simulink model "clearing_faulted_segment_travelling_Wave"  (R2018a)
settings: Solver=ode23t  StartTime=0.0  StopTime=2  MaxStep=1e-3  RelTol=1e-3
values from neighbouring files (symbols this model uses):
  AC_lim = [1.5 -1.5]    [MT_HVDC_initialize.m]
  C_pm = 10.48e-3    (= 0.01048)    [MT_HVDC_initialize.m]
  ccsc_lim = [1.0 -1.0]    [MT_HVDC_initialize.m]
  DC_lim = [1.05 -1.05]    [MT_HVDC_initialize.m]
  f = 50    [MT_HVDC_initialize.m]
  Fc = 50    [MT_HVDC_initialize.m]
  Fn_filter = 1000    [MT_HVDC_initialize.m]
  Ireg_lim_i = [1.5, -1.5]    [MT_HVDC_initialize.m]
  Ireg_lim_r = [1.5, -1.5]    [MT_HVDC_initialize.m]
  Ki_ACreg_i = 260    [MT_HVDC_initialize.m]
  Ki_ccsc = 5    [MT_HVDC_initialize.m]
  Ki_DCreg_r = 150    [MT_HVDC_initialize.m]
  Ki_Ireg_i = 200    [MT_HVDC_initialize.m]
  Ki_Ireg_r = 100    [MT_HVDC_initialize.m]
  Ki_R_inv = 150000    [MT_HVDC_initialize.m]
  Ki_R_rec = 5000    [MT_HVDC_initialize.m]
  Kp_ACreg_i = 2    [MT_HVDC_initialize.m]
  Kp_ccsc = 1    [MT_HVDC_initialize.m]
  Kp_DCreg_r = 8    [MT_HVDC_initialize.m]
  Kp_Ireg_i = 2    [MT_HVDC_initialize.m]
  Kp_Ireg_r = 2    [MT_HVDC_initialize.m]
  Kp_R_inv = 0.001    [MT_HVDC_initialize.m]
  Kp_R_rec = 0.001    [MT_HVDC_initialize.m]
  L1_pu = 0.109    [MT_HVDC_initialize.m]
  L2_pu = 0.0824    [MT_HVDC_initialize.m]
  L_arm = L_arm_pu*Z_base66/w    [MT_HVDC_initialize.m]
  L_arm_pu = 0.15    [MT_HVDC_initialize.m]
  L_int = X_int/w    [MT_HVDC_initialize.m]
  n = 50    [MT_HVDC_initialize.m]
  n2 = 50    [MT_HVDC_initialize.m]
  P_nom = 220e6    (= 220000000)    [MT_HVDC_initialize.m]
  R1_pu = 0.00206    [MT_HVDC_initialize.m]
  R2_pu = 0.00206    [MT_HVDC_initialize.m]
  R_arm = 0.03    [MT_HVDC_initialize.m]
  R_arm_pu = R_arm/Z_base66    [MT_HVDC_initialize.m]
  R_int = sqrt((z_int_400^2)/(1+xr_ratio^2))    [MT_HVDC_initialize.m]
  Rg_T1 = 40    [MT_HVDC_initialize.m]
  S1_nom = P_nom    (= 220000000)    [MT_HVDC_initialize.m]
  S2_nom = P_nom    (= 220000000)    [MT_HVDC_initialize.m]
  T_fault = 1.4    [MT_HVDC_initialize.m]
  Ts_Control = 40e-6    (= 4e-05)    [MT_HVDC_initialize.m]
  Ts_Power = 20e-6    (= 2e-05)    [MT_HVDC_initialize.m]
  V1_prim = V_prim    (= 400000)    [MT_HVDC_initialize.m]
  V1_sec = V_grid    (= 66000)    [MT_HVDC_initialize.m]
  V2_prim = V_grid    (= 66000)    [MT_HVDC_initialize.m]
  V2_sec = 18e3    (= 18000)    [MT_HVDC_initialize.m]
  V_ac_ref = 1.035    [MT_HVDC_initialize.m]
  V_grid = 66e3    (= 66000)    [MT_HVDC_initialize.m]
  V_prim = 400e3    (= 400000)    [MT_HVDC_initialize.m]
  Vc_pm_r = 0*Vdc_nom/n    (= 0)    [MT_HVDC_initialize.m]
  Vdc_nom = 135e3    (= 135000)    [MT_HVDC_initialize.m]
  w = 2*pi*f    (= 314.159265359)    [MT_HVDC_initialize.m]
  z0z1 = 0.8    [MT_HVDC_initialize.m]
  Zeta_filter = 1    [MT_HVDC_initialize.m]
undefined symbols (not defined in the file or in its folder): D1, Delta, DiscIntNeverNeededParam
libraries: powerlib x417, powerlib_meascontrol x130, simulink x84, powerlib_extras x8, simulink_extras x5
(part 1 of 17)
settings Model: SimulationMode=accelerator  NumberOfSteps=1000  SnapshotBufferSize=5000  SnapshotInterval=100  Creator=tslettba  LastModifiedBy=eslam
settings SolverCC: AlgebraicLoopSolver=LineSearch  DecoupledContinuousIntegration=on
settings OptimizationCC: BooleanDataType=off  EfficientMapNaN2IntZero=off
settings DebuggingCC: UnconnectedLineMsg=none
settings HardwareCC: TargetBitPerPointer=64  TargetBitPerSizeT=64  TargetBitPerPtrDiffT=64  TargetLongLongMode=on  TargetIntDivRoundTo=Zero  TargetEndianess=LittleEndian  TargetWordSize=64  TargetHWDeviceType=MATLAB Host  ProdEqTarget=off
settings ModelReferenceCC: ModelReferenceMinAlgLoopOccurrences=on
settings CodeAppCC: MaxIdLength=128
settings GRTTargetCC: TargetLangStandard=C89/C90 (ANSI)  CombineOutputUpdateFcns=off  GRTInterface=on
settings SimscapeCC: SimscapeNormalizeSystem=off

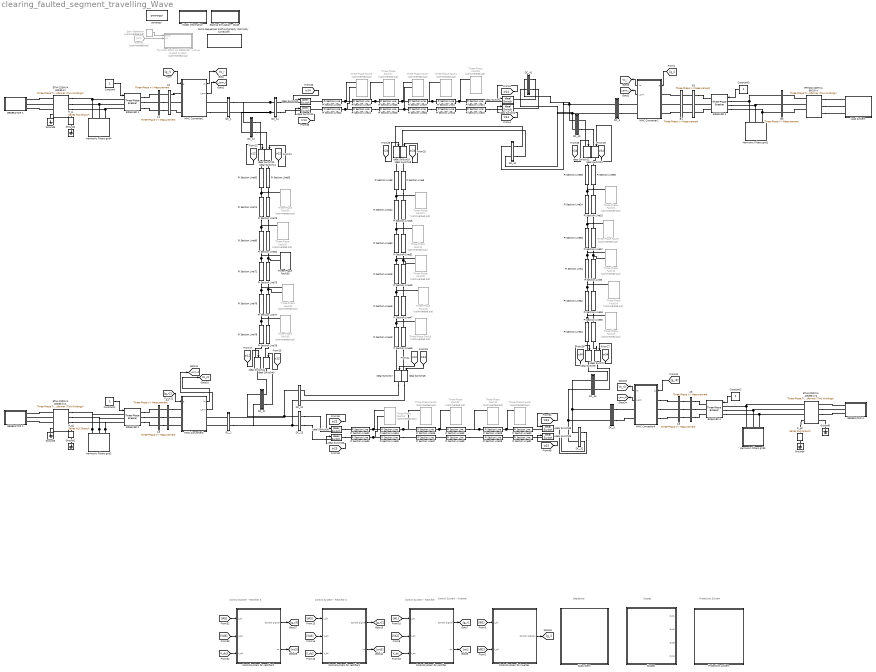
== system clearing_faulted_segment_travelling_Wave ==
  note: Protection System
  note: Scopes
  note: Control System - Inverter
  note: Control System - Rectifier
  note: Sequencer
  note: Control System - Rectifier 2
  note: Control System - Rectifier 3
  " " : powerlib_meascontrol/Pulse & Signal Generators/Stair Generator  Commented=on  t=[0, 999]  e=[1,0]  Ts=0
      settings: SourceProductName=Simscape Electrical
  " R_g" : powerlib/Elements/Series RLC Branch  LConnTagsString=__new0  RConnTagsString=__new0  BranchType=R  Resistance=Rg_T1  Inductance=1e-3  SetiL0=off  InitialCurrent=0  Capacitance=1e-6  Setx0=off  InitialVoltage=0  Measurements=None
      settings: SourceProductName=Simscape Electrical
  " R_g1" : powerlib/Elements/Series RLC Branch  LConnTagsString=__new0  RConnTagsString=__new0  BranchType=R  Resistance=Rg_T1  Inductance=1e-3  SetiL0=off  InitialCurrent=0  Capacitance=1e-6  Setx0=off  InitialVoltage=0  Measurements=None
      settings: SourceProductName=Simscape Electrical
  " R_g2" : powerlib/Elements/Series RLC Branch  LConnTagsString=__new0  RConnTagsString=__new0  BranchType=R  Resistance=Rg_T1  Inductance=1e-3  SetiL0=off  InitialCurrent=0  Capacitance=1e-6  Setx0=off  InitialVoltage=0  Measurements=None
      settings: SourceProductName=Simscape Electrical
  A1 : powerlib/Measurements/Three-Phase V-I Measurement  VoltageMeasurement=phase-to-phase  SetLabelV=on  LabelV=VA1  Vpu=off  VpuLL=off  CurrentMeasurement=yes  SetLabelI=on  LabelI=IA1  Ipu=off  Pbase=100e6  Vbase=500e3  OutputType=Complex  PhasorSimulation=off  PSBequivalent=0
      settings: SourceProductName=Simscape Electrical
  A2 : powerlib/Measurements/Three-Phase V-I Measurement  VoltageMeasurement=phase-to-ground  SetLabelV=on  LabelV=VA2  Vpu=off  VpuLL=off  CurrentMeasurement=no  SetLabelI=on  LabelI=IA2  Ipu=off  Pbase=100e6  Vbase=500e3  OutputType=Complex  PhasorSimulation=off  PSBequivalent=0
      settings: SourceProductName=Simscape Electrical
  A3 : powerlib/Measurements/Three-Phase V-I Measurement  VoltageMeasurement=phase-to-phase  SetLabelV=on  LabelV=VA3  Vpu=off  VpuLL=off  CurrentMeasurement=yes  SetLabelI=on  LabelI=IA3  Ipu=off  Pbase=100e6  Vbase=500e3  OutputType=Complex  PhasorSimulation=off  PSBequivalent=0
      settings: SourceProductName=Simscape Electrical
  A4 : powerlib/Measurements/Three-Phase V-I Measurement  VoltageMeasurement=phase-to-ground  SetLabelV=on  LabelV=VA4  Vpu=off  VpuLL=off  CurrentMeasurement=no  SetLabelI=on  LabelI=IA2  Ipu=off  Pbase=100e6  Vbase=500e3  OutputType=Complex  PhasorSimulation=off  PSBequivalent=0
      settings: SourceProductName=Simscape Electrical
  A5 : powerlib/Measurements/Three-Phase V-I Measurement  VoltageMeasurement=phase-to-phase  SetLabelV=on  LabelV=VA5  Vpu=off  VpuLL=off  CurrentMeasurement=yes  SetLabelI=on  LabelI=IA5  Ipu=off  Pbase=100e6  Vbase=500e3  OutputType=Complex  PhasorSimulation=off  PSBequivalent=0
      settings: SourceProductName=Simscape Electrical
  A6 : powerlib/Measurements/Three-Phase V-I Measurement  VoltageMeasurement=phase-to-ground  SetLabelV=on  LabelV=VA6  Vpu=off  VpuLL=off  CurrentMeasurement=no  SetLabelI=on  LabelI=IA2  Ipu=off  Pbase=100e6  Vbase=500e3  OutputType=Complex  PhasorSimulation=off  PSBequivalent=0
      settings: SourceProductName=Simscape Electrical
  B1 : powerlib/Measurements/Three-Phase V-I Measurement  VoltageMeasurement=phase-to-phase  SetLabelV=on  LabelV=VB1  Vpu=off  VpuLL=off  CurrentMeasurement=yes  SetLabelI=on  LabelI=IB1  Ipu=off  Pbase=100e6  Vbase=500e3  OutputType=Complex  PhasorSimulation=off  PSBequivalent=0
      settings: SourceProductName=Simscape Electrical
  B2 : powerlib/Measurements/Three-Phase V-I Measurement  VoltageMeasurement=phase-to-ground  SetLabelV=on  LabelV=VB2  Vpu=off  VpuLL=off  CurrentMeasurement=no  SetLabelI=on  LabelI=IB1  Ipu=off  Pbase=100e6  Vbase=500e3  OutputType=Complex  PhasorSimulation=off  PSBequivalent=0
      settings: SourceProductName=Simscape Electrical
  B3 : powerlib/Measurements/Three-Phase V-I Measurement  VoltageMeasurement=phase-to-ground  SetLabelV=on  LabelV=VB3  Vpu=off  VpuLL=off  CurrentMeasurement=yes  SetLabelI=on  LabelI=IB3  Ipu=off  Pbase=100e6  Vbase=500e3  OutputType=Complex  PhasorSimulation=off  PSBequivalent=0
      settings: SourceProductName=Simscape Electrical
  BREAKER {1..4} (4 alike) : powerlib/Elements/Three-Phase Breaker  InitialState=closed  SwitchA=on  SwitchB=on  SwitchC=on  SwitchTimes=[30/60]*10000  External=on  BreakerResistance=0.001  SnubberResistance=1e6  SnubberCapacitance=inf  Measurements=None
      settings: SourceProductName=Simscape Electrical
  Constant{,1..3} (4 alike) : Constant
  Controlsystem for Inverter : Subsystem  Variant=on  VariantControl=Variant1  OverrideUsingVariant=Variant1
  Controlsystem for rectifier : Subsystem  Variant=on  VariantControl=Variant1  OverrideUsingVariant=Variant1
  Controlsystem for rectifier1 : Subsystem  Variant=on  VariantControl=Variant1  OverrideUsingVariant=Variant1
  Controlsystem for rectifier2 : Subsystem  Variant=on  VariantControl=Variant1  OverrideUsingVariant=Variant1
  DC_1 : Subsystem
  DC_12 : Subsystem
  DC_14 : Subsystem
  DC_2 : Subsystem
  DC_21 : Subsystem
  DC_23 : Subsystem
  DC_24 : Subsystem
  DC_3 : Subsystem
  DC_32 : Subsystem
  DC_34 : Subsystem
  DC_4 : Subsystem
  DC_41 : Subsystem
  DC_42 : Subsystem
  DC_43 : Subsystem
  ETH102 220MVA 66/18 kV : powerlib/Elements/Three-Phase Transformer (Two Windings)  Winding1Connection=Yn  Winding2Connection=Delta (D1)  CoreType=Three single-phase transformers  SetSaturation=off  Hysteresis=off  DataFile='hysteresis'  SetInitialFlux=off  Measurements=None  UNITS=pu  NominalPower=[S2_nom , f ]  Winding1=[V2_prim , R2_pu*0.5 , L2_pu*0.5]  Winding2=[V2_sec , R2_pu*0.5 , L2_pu*0.5]  Rm=500  Lm=500  L0=0.5  Saturation="[ 0,0  ;  0.005,1.2  ;  1.0,1.4 ]"  InitialFluxes=[ 0.8 , -0.8 , 0.7 ]  MoreParameters=off  BreakLoop=off  DataType=off  TransfoNumber=0
      settings: SourceProductName=Simscape Electrical
  ETH4 220MVA 400/66 kV : powerlib/Elements/Three-Phase Transformer (Two Windings)  Winding1Connection=Yn  Winding2Connection=Yn  CoreType=Three single-phase transformers  SetSaturation=off  Hysteresis=off  DataFile='hysteresis'  SetInitialFlux=off  Measurements=None  UNITS=pu  NominalPower=[S1_nom , f ]  Winding1=[V1_prim , R1_pu*0.5, L1_pu*0.5]  Winding2=[V1_sec , R1_pu*0.5, L1_pu*0.5]  Rm=500  Lm=500  L0=0.5  Saturation="[ 0,0  ;  0.005,1.2  ;  1.0,1.4 ]"  InitialFluxes=[ 0.8 , -0.8 , 0.7 ]  MoreParameters=off  BreakLoop=off  DataType=off  TransfoNumber=0
      settings: SourceProductName=Simscape Electrical
  ETH4 220MVA 400/66 kV1 : powerlib/Elements/Three-Phase Transformer (Two Windings)  Winding1Connection=Yn  Winding2Connection=Yn  CoreType=Three single-phase transformers  SetSaturation=off  Hysteresis=off  DataFile='hysteresis'  SetInitialFlux=off  Measurements=None  UNITS=pu  NominalPower=[S1_nom , f ]  Winding1=[V1_prim , R1_pu*0.5, L1_pu*0.5]  Winding2=[V1_sec , R1_pu*0.5, L1_pu*0.5]  Rm=500  Lm=500  L0=0.5  Saturation="[ 0,0  ;  0.005,1.2  ;  1.0,1.4 ]"  InitialFluxes=[ 0.8 , -0.8 , 0.7 ]  MoreParameters=off  BreakLoop=off  DataType=off  TransfoNumber=0
      settings: SourceProductName=Simscape Electrical
  ETH4 220MVA 400/66 kV2 : powerlib/Elements/Three-Phase Transformer (Two Windings)  Winding1Connection=Yn  Winding2Connection=Yn  CoreType=Three single-phase transformers  SetSaturation=off  Hysteresis=off  DataFile='hysteresis'  SetInitialFlux=off  Measurements=None  UNITS=pu  NominalPower=[S1_nom , f ]  Winding1=[V1_prim , R1_pu*0.5, L1_pu*0.5]  Winding2=[V1_sec , R1_pu*0.5, L1_pu*0.5]  Rm=500  Lm=500  L0=0.5  Saturation="[ 0,0  ;  0.005,1.2  ;  1.0,1.4 ]"  InitialFluxes=[ 0.8 , -0.8 , 0.7 ]  MoreParameters=off  BreakLoop=off  DataType=off  TransfoNumber=0
      settings: SourceProductName=Simscape Electrical
  Extra Sequences and functionality (Normally turned off) : Subsystem
  From11 : From  Commented=on  GotoTag=wt
  GENERATOR 1 : Subsystem  mask{V_g=V_prim*1.03, F_s=f, R=R_int, L=L_int, T1=9999, T2=0.075, A=-0.5, BC=-0.5}
      mask prompts: V_g "Voltage (line-line RMS)"; F_s "Frequency:"; R "Internal Resistance:"; L "Internal inductance:"; T1 "Fault start:"; T2 "Fault duration:"; A "Phase A magnitude change:"; BC "Phase B,C magnitude change:"
      mask DialogControl DescTextVar Prompt: This block simulates a fully controllable Grid equivalent with internal parameters. It is possible to program voltage dips/swells for one, two or three phases.
      mask DialogControl asd Prompt: Source parameters:
      mask DialogControl Control3 Prompt: Fault simulation:
  GENERATOR 2 : Subsystem  mask{V_g=V_prim*1.03, F_s=f, R=R_int, L=L_int, T1=9999, T2=0.075, A=-0.5, BC=-0.5}
      mask prompts: V_g "Voltage (line-line RMS)"; F_s "Frequency:"; R "Internal Resistance:"; L "Internal inductance:"; T1 "Fault start:"; T2 "Fault duration:"; A "Phase A magnitude change:"; BC "Phase B,C magnitude change:"
      mask DialogControl DescTextVar Prompt: This block simulates a fully controllable Grid equivalent with internal parameters. It is possible to program voltage dips/swells for one, two or three phases.
      mask DialogControl asd Prompt: Source parameters:
      mask DialogControl Control3 Prompt: Fault simulation:
  GENERATOR 3 : Subsystem  mask{V_g=V_prim*1.03, F_s=f, R=R_int, L=L_int, T1=9999, T2=0.075, A=-0.5, BC=-0.5}
      mask prompts: V_g "Voltage (line-line RMS)"; F_s "Frequency:"; R "Internal Resistance:"; L "Internal inductance:"; T1 "Fault start:"; T2 "Fault duration:"; A "Phase A magnitude change:"; BC "Phase B,C magnitude change:"
      mask DialogControl DescTextVar Prompt: This block simulates a fully controllable Grid equivalent with internal parameters. It is possible to program voltage dips/swells for one, two or three phases.
      mask DialogControl asd Prompt: Source parameters:
      mask DialogControl Control3 Prompt: Fault simulation:
  Ground{1..6} (6 alike) : powerlib/Elements/Ground  LConnTagsString=a
      settings: SourceProductName=Simscape Electrical
  Harmonic Filters grid1 : Subsystem
      mask Display: disp('Harmonic Filters')
  Harmonic Filters grid2 : Subsystem
      mask Display: disp('Harmonic Filters')
  Harmonic Filters grid3 : Subsystem
      mask Display: disp('Harmonic Filters')
  Harmonic Filters grid4 : Subsystem
      mask Display: disp('Harmonic Filters')
  Ideal Switch{2,4,7,9..11,14..20,23,29..30,33,38,40..41} (20 alike) : powerlib/Power Electronics/Ideal Switch  Ron=0.001  Lon=0  IC=1  Rs=1e5  Cs=inf  Measurements=off
      settings: SourceProductName=Simscape Electrical
  Load System : Subsystem
      mask Display: disp('Load')
  MMC Converter1 : Subsystem
  MMC Converter2 : Subsystem
  MMC Converter3 : Subsystem
  MMC Converter4 : Subsystem
  Model Information : Subsystem
  Pi Section Line{1,4..5,8..11,14..15,18..39,44..59,72..84} (60 alike) : powerlib/Elements/Pi Section Line  LConnTagsString=__new0  RConnTagsString=__new0  Frequency=50  Resistance=0.01273  Inductance=0.9337e-3  Capacitance=12.74e-18  Length=25  PiSections=1  Measurements=None
      settings: AttributesFormatString=\n  SourceProductName=Simscape Electrical  SourceProductBaseCode=PS
  Protection system : Subsystem
  "Scopes " : Subsystem
  Startup Simulation - Guide : Subsystem
  Subsystem : Subsystem
  Three-Phase Fault{1,3,5,8..10,12..14,16..17,21..23,25} (15 alike) : powerlib/Elements/Three-Phase Fault  Commented=on  InitialStates=0  FaultA=on  FaultB=off  FaultC=off  GroundFault=on  SwitchTimes=0.7  External=off  SwitchStatus=NaN  FaultResistance=1  GroundResistance=1  SnubberResistance=1e6  SnubberCapacitance=inf  Measurements=Fault voltages and currents
      settings: SourceProductName=Simscape Electrical
  Three-Phase Fault15 : powerlib/Elements/Three-Phase Fault  Commented=on  InitialStates=0  FaultA=on  FaultB=off  FaultC=off  GroundFault=on  SwitchTimes=0.7  External=off  SwitchStatus=NaN  FaultResistance=0.1  GroundResistance=1  SnubberResistance=1e6  SnubberCapacitance=inf  Measurements=Fault voltages and currents
      settings: SourceProductName=Simscape Electrical
  Three-Phase Fault20 : powerlib/Elements/Three-Phase Fault  Commented=on  InitialStates=0  FaultA=off  FaultB=on  FaultC=off  GroundFault=on  SwitchTimes=0.7  External=off  SwitchStatus=NaN  FaultResistance=0.1  GroundResistance=1  SnubberResistance=1e6  SnubberCapacitance=inf  Measurements=Fault voltages and currents
      settings: SourceProductName=Simscape Electrical
  Three-Phase Fault24 : powerlib/Elements/Three-Phase Fault  Commented=on  InitialStates=0  FaultA=on  FaultB=off  FaultC=off  GroundFault=on  SwitchTimes=0.7  External=off  SwitchStatus=NaN  FaultResistance=0.1  GroundResistance=1  SnubberResistance=1e6  SnubberCapacitance=inf  Measurements=Fault voltages and currents
      settings: SourceProductName=Simscape Electrical
  Three-Phase Fault26 : powerlib/Elements/Three-Phase Fault  Commented=on  InitialStates=0  FaultA=on  FaultB=off  FaultC=off  GroundFault=on  SwitchTimes=1.5  External=off  SwitchStatus=NaN  FaultResistance=1  GroundResistance=1  SnubberResistance=1e6  SnubberCapacitance=inf  Measurements=Fault voltages and currents
      settings: SourceProductName=Simscape Electrical
  Three-Phase Fault32 : powerlib/Elements/Three-Phase Fault  Commented=on  InitialStates=0  FaultA=on  FaultB=off  FaultC=off  GroundFault=on  SwitchTimes=0.6  External=off  SwitchStatus=NaN  FaultResistance=0.1  GroundResistance=1  SnubberResistance=1e6  SnubberCapacitance=inf  Measurements=Fault voltages and currents
      settings: SourceProductName=Simscape Electrical
  Three-Phase Fault33 : powerlib/Elements/Three-Phase Fault  InitialStates=0  FaultA=on  FaultB=on  FaultC=off  GroundFault=on  SwitchTimes=1.5  External=off  SwitchStatus=NaN  FaultResistance=0.1  GroundResistance=1  SnubberResistance=1e6  SnubberCapacitance=inf  Measurements=Fault voltages and currents
      settings: SourceProductName=Simscape Electrical
  Three-Phase Fault34 : powerlib/Elements/Three-Phase Fault  Commented=on  InitialStates=0  FaultA=on  FaultB=off  FaultC=off  GroundFault=on  SwitchTimes=0.6  External=off  SwitchStatus=NaN  FaultResistance=1  GroundResistance=1  SnubberResistance=1e6  SnubberCapacitance=inf  Measurements=Fault voltages and currents
      settings: SourceProductName=Simscape Electrical
  Three-Phase Fault35 : powerlib/Elements/Three-Phase Fault  Commented=on  InitialStates=0  FaultA=on  FaultB=off  FaultC=off  GroundFault=on  SwitchTimes=0.6  External=off  SwitchStatus=NaN  FaultResistance=0.1  GroundResistance=1  SnubberResistance=1e6  SnubberCapacitance=inf  Measurements=Fault voltages and currents
      settings: SourceProductName=Simscape Electrical
  Three-Phase Fault6 : powerlib/Elements/Three-Phase Fault  Commented=on  InitialStates=0  FaultA=on  FaultB=off  FaultC=off  GroundFault=on  SwitchTimes=0.7  External=off  SwitchStatus=NaN  FaultResistance=0.1  GroundResistance=1  SnubberResistance=1e6  SnubberCapacitance=inf  Measurements=Fault voltages and currents
      settings: SourceProductName=Simscape Electrical
  Three-Phase Fault7 : powerlib/Elements/Three-Phase Fault  Commented=on  InitialStates=0  FaultA=off  FaultB=on  FaultC=off  GroundFault=on  SwitchTimes=0.6  External=off  SwitchStatus=NaN  FaultResistance=1  GroundResistance=1  SnubberResistance=1e6  SnubberCapacitance=inf  Measurements=Fault voltages and currents
      settings: SourceProductName=Simscape Electrical
  Thyristor Static AC BREAKER - Active bypass system : Subsystem  Commented=on
  powergui : powerlib/powergui  Priority=1  SimulationMode=Discrete  SampleTime=Ts_Power  frequency=60  Iterations=50  frequencyindice=0  Pbase=100e6  ErrMax=1e-4  UnitsV=kV  UnitsW=MW  buscounter=0  FunctionMessages=off  echomessages=off  EnableUseOfTLC=off  CurrentSourceSwitches=off  DisableSnubberDevices=off  DisableRonSwitches=off  DisableVfSwitches=off  DisplayEquations=off  SolverType=Tustin/Backward Euler (TBE)  Interpol=off  ExternalGateDelay=off  methode=off  Ts=100  x0status=blocks  SPID=on  SwTol=0  HookPort=off  RestoreLinks=warning  ResistiveCurrentMeasurement=off  Frange=[0:10:1000000]  Ylog=off  Xlog=on  ShowGrid=on  save=off  variable=ZData  structure=I_inv  ZoomFFT=off  StartTime=2  cycles=1  DisplayStyle=1  fundamental=50  FreqAxis=on  MaxFrequency=3000  frequencyindicesteady=1  RmsSteady=1  display=off
  tag scope: I_arm_i=global, I_arm_r2=global, I_arm_r3=global, I_arm_r=global, Vc_i=global, Vc_r2=global, Vc_r3=global, Vc_r=global
  wires:
  [g_i] -> MMC Converter2/1(g)
  MMC Converter1/1(Vc) -> [Vc_r]
  MMC Converter1/2(I_arm) -> [I_arm_r]
  MMC Converter2/2(I_arm) -> [I_arm_i]
  MMC Converter2/1(Vc) -> [Vc_i]
  [g_r] -> MMC Converter1/1(g)
  Controlsystem for Inverter/1(" Control Signal1") -> [g_i]
  [VB2] -> Controlsystem for Inverter/2("V_ph ")
  [IB1] -> Controlsystem for Inverter/1("I_ph ")
  [IA1] -> Controlsystem for rectifier/1("I_ph ")
  [VA2] -> Controlsystem for rectifier/2("V_ph ")
  [V_dc] -> Controlsystem for rectifier/3("V_dc ")
  Controlsystem for rectifier/1(" Control Signal") -> [g_r]
  " "/1 -> Thyristor Static AC BREAKER - Active bypass system/1(Block)
  Controlsystem for rectifier/2(" wt") -> [wt]
  From11/1 -> Thyristor Static AC BREAKER - Active bypass system/2(wt)
  Constant/1 -> BREAKER 1/1
  MMC Converter3/2(I_arm) -> [I_arm_r2]
  Constant1/1 -> BREAKER 2/1
  MMC Converter3/1(Vc) -> [Vc_r2]
  [g_r2] -> MMC Converter3/1(g)
  [IA3] -> Controlsystem for rectifier1/1("I_ph ")
  [VA4] -> Controlsystem for rectifier1/2("V_ph ")
  [V_dc2] -> Controlsystem for rectifier1/3("V_dc ")
  Controlsystem for rectifier1/2(" wt") -> [wt2]
  Controlsystem for rectifier1/1(" Control Signal") -> [g_r2]
  Constant2/1 -> BREAKER 3/1
  [g_r3] -> MMC Converter4/1(g)
  MMC Converter4/2(I_arm) -> [I_arm_r3]
  MMC Converter4/1(Vc) -> [Vc_r3]
  Controlsystem for rectifier2/1(" Control Signal") -> [g_r3]
  Controlsystem for rectifier2/2(" wt") -> [wt3]
  [V_dc3] -> Controlsystem for rectifier2/3("V_dc ")
  [VA6] -> Controlsystem for rectifier2/2("V_ph ")
  [IA5] -> Controlsystem for rectifier2/1("I_ph ")
  Constant3/1 -> BREAKER 4/1
  [tr14] -> Ideal Switch2/1
  [tr34] -> Ideal Switch10/1
  [tr34] -> Ideal Switch11/1
  [tr14] -> Ideal Switch4/1
  [tr24] -> Ideal Switch18/1
  [tr34] -> Ideal Switch7/1
  [tr12] -> Ideal Switch14/1
  [tr24] -> Ideal Switch16/1
  [tr34] -> Ideal Switch9/1
  [tr12] -> Ideal Switch41/1
  [tr14] -> Ideal Switch23/1
  [tr23] -> Ideal Switch33/1
  [tr23] -> Ideal Switch30/1
  [tr24] -> Ideal Switch19/1
  [tr12] -> Ideal Switch15/1
  [tr23] -> Ideal Switch38/1
  [tr23] -> Ideal Switch29/1
  [tr14] -> Ideal Switch20/1
  [tr12] -> Ideal Switch40/1
  [tr24] -> Ideal Switch17/1
  connections:
  B2/LConn3 -- B1/RConn3
  B2/LConn2 -- B1/RConn2
  B2/LConn1 -- B1/RConn1
  DC_1/LConn1 -- MMC Converter1/RConn1
  B1/LConn3 -- MMC Converter2/LConn3
  BREAKER 1/RConn3 -- A1/LConn3
  BREAKER 1/RConn1 -- A1/LConn1
  BREAKER 1/RConn2 -- A1/LConn2
  A2/LConn1 -- A1/RConn1
  A1/RConn2 -- A2/LConn2
  A1/RConn3 -- A2/LConn3
  MMC Converter1/LConn3 -- A2/RConn3
  MMC Converter1/LConn2 -- A2/RConn2
  B3/LConn1 -- BREAKER 4/LConn1 -- Harmonic Filters grid1/LConn1
  B3/LConn3 -- BREAKER 4/LConn3 -- Harmonic Filters grid1/LConn3
  B3/LConn2 -- BREAKER 4/LConn2 -- Harmonic Filters grid1/LConn2
  ETH102 220MVA 66/18 kV/RConn1 -- Load System/LConn1
  ETH102 220MVA 66/18 kV/RConn3 -- Load System/LConn3
  ETH4 220MVA 400/66 kV/RConn3 -- BREAKER 1/LConn3 -- Harmonic Filters grid4/LConn3
  ETH4 220MVA 400/66 kV/RConn2 -- BREAKER 1/LConn2 -- Harmonic Filters grid4/LConn2
  ETH4 220MVA 400/66 kV/RConn1 -- BREAKER 1/LConn1 -- Harmonic Filters grid4/LConn1
  B1/LConn1 -- MMC Converter2/LConn1
  B1/LConn2 -- MMC Converter2/LConn2
  ETH102 220MVA 66/18 kV/RConn2 -- Load System/LConn2
  ETH102 220MVA 66/18 kV/LConn2 -- B3/RConn2
  ETH102 220MVA 66/18 kV/LConn3 -- B3/RConn3
  ETH102 220MVA 66/18 kV/LConn1 -- B3/RConn1
  ETH4 220MVA 400/66 kV/LConn2 -- GENERATOR 1/RConn2
  ETH4 220MVA 400/66 kV/LConn1 -- GENERATOR 1/RConn1
  ETH4 220MVA 400/66 kV/LConn3 -- GENERATOR 1/RConn3
  Ground2/LConn1 -- " R_g"/RConn1
  Ground5/LConn1 -- ETH4 220MVA 400/66 kV/LConn4
  ETH4 220MVA 400/66 kV/RConn4 -- " R_g"/LConn1
  A2/RConn1 -- MMC Converter1/LConn1
  Harmonic Filters grid2/LConn1 -- ETH4 220MVA 400/66 kV1/RConn1 -- BREAKER 2/LConn1
  Harmonic Filters grid2/LConn2 -- BREAKER 2/LConn2 -- ETH4 220MVA 400/66 kV1/RConn2
  Harmonic Filters grid2/LConn3 -- BREAKER 2/LConn3 -- ETH4 220MVA 400/66 kV1/RConn3
  MMC Converter3/LConn2 -- A4/RConn2
  ETH4 220MVA 400/66 kV1/LConn1 -- GENERATOR 2/RConn1
  BREAKER 2/RConn2 -- A3/LConn2
  A4/RConn1 -- MMC Converter3/LConn1
  ETH4 220MVA 400/66 kV1/LConn2 -- GENERATOR 2/RConn2
  Ground1/LConn1 -- " R_g1"/RConn1
  BREAKER 2/RConn3 -- A3/LConn3
  ETH4 220MVA 400/66 kV1/RConn4 -- " R_g1"/LConn1
  Ground3/LConn1 -- ETH4 220MVA 400/66 kV1/LConn4
  A3/RConn2 -- A4/LConn2
  ETH4 220MVA 400/66 kV1/LConn3 -- GENERATOR 2/RConn3
  BREAKER 2/RConn1 -- A3/LConn1
  A4/LConn1 -- A3/RConn1
  MMC Converter3/LConn3 -- A4/RConn3
  A3/RConn3 -- A4/LConn3
  Ground4/LConn1 -- " R_g2"/RConn1
  MMC Converter4/LConn1 -- A5/RConn1
  MMC Converter4/LConn2 -- A5/RConn2
  MMC Converter4/LConn3 -- A5/RConn3
  A6/LConn1 -- BREAKER 3/RConn1
  A6/LConn2 -- BREAKER 3/RConn2
  A6/LConn3 -- BREAKER 3/RConn3
  Harmonic Filters grid3/LConn1 -- ETH4 220MVA 400/66 kV2/RConn1 -- BREAKER 3/LConn1
  BREAKER 3/LConn2 -- ETH4 220MVA 400/66 kV2/RConn2 -- Harmonic Filters grid3/LConn2
  BREAKER 3/LConn3 -- Harmonic Filters grid3/LConn3 -- ETH4 220MVA 400/66 kV2/RConn3
  GENERATOR 3/RConn1 -- ETH4 220MVA 400/66 kV2/LConn1
  ETH4 220MVA 400/66 kV2/LConn2 -- GENERATOR 3/RConn2
  ETH4 220MVA 400/66 kV2/LConn3 -- GENERATOR 3/RConn3
  Ground6/LConn1 -- ETH4 220MVA 400/66 kV2/LConn4
  " R_g2"/LConn1 -- ETH4 220MVA 400/66 kV2/RConn4
  A5/LConn1 -- A6/RConn1
  A5/LConn2 -- A6/RConn2
  A5/LConn3 -- A6/RConn3
  DC_2/LConn2 -- MMC Converter3/RConn2
  DC_4/RConn2 -- MMC Converter2/RConn2
  MMC Converter1/RConn2 -- DC_1/LConn2
  DC_4/RConn1 -- MMC Converter2/RConn1
  DC_2/LConn1 -- MMC Converter3/RConn1
  DC_3/LConn1 -- MMC Converter4/RConn1
  DC_3/LConn2 -- MMC Converter4/RConn2
  B2/RConn1 -- BREAKER 4/RConn1
  BREAKER 4/RConn2 -- B2/RConn2
  BREAKER 4/RConn3 -- B2/RConn3
  Pi Section Line50/RConn1 -- Three-Phase Fault12/LConn1 -- Pi Section Line44/LConn1
  DC_14/LConn2 -- DC_12/LConn2 -- DC_1/RConn2
  Pi Section Line28/RConn1 -- Pi Section Line30/LConn1 -- Three-Phase Fault8/LConn1
  Pi Section Line4/RConn1 -- Three-Phase Fault15/LConn1 -- Pi Section Line56/LConn1
  Pi Section Line32/RConn1 -- Pi Section Line34/LConn1 -- Three-Phase Fault24/LConn1
  Pi Section Line73/RConn1 -- Three-Phase Fault33/LConn2 -- Pi Section Line81/LConn1
  Pi Section Line25/RConn1 -- Three-Phase Fault7/LConn1 -- Pi Section Line27/LConn1
  Pi Section Line21/RConn1 -- Three-Phase Fault6/LConn1 -- Pi Section Line23/LConn1
  Pi Section Line52/RConn1 -- Pi Section Line4/LConn1 -- Three-Phase Fault14/LConn1
  Pi Section Line33/RConn1 -- Pi Section Line35/LConn1 -- Three-Phase Fault24/LConn2
  Pi Section Line28/LConn1 -- Pi Section Line38/RConn1 -- Three-Phase Fault10/LConn1
  Pi Section Line22/RConn1 -- Pi Section Line24/LConn1 -- Three-Phase Fault6/LConn2
  DC_24/LConn2 -- DC_23/LConn2 -- DC_21/LConn2 -- DC_2/RConn2
  Pi Section Line36/RConn1 -- Pi Section Line38/LConn1 -- Three-Phase Fault25/LConn1
  Pi Section Line1/RConn1 -- Three-Phase Fault16/LConn1 -- Pi Section Line11/LConn1
  Pi Section Line76/RConn1 -- Pi Section Line72/LConn1 -- Three-Phase Fault32/LConn1
  Pi Section Line48/RConn1 -- Pi Section Line46/LConn1 -- Three-Phase Fault5/LConn1
  Pi Section Line54/RConn1 -- Three-Phase Fault23/LConn1 -- Pi Section Line52/LConn1
  Pi Section Line74/RConn1 -- Three-Phase Fault34/LConn1 -- Pi Section Line82/LConn1
  Pi Section Line34/RConn1 -- Three-Phase Fault9/LConn1 -- Pi Section Line36/LConn1
  DC_34/LConn2 -- DC_3/RConn2 -- DC_32/LConn2
  Pi Section Line23/RConn1 -- Pi Section Line25/LConn1 -- Three-Phase Fault17/LConn1
  Pi Section Line80/RConn1 -- Pi Section Line74/LConn1 -- Three-Phase Fault26/LConn1
  Pi Section Line46/RConn1 -- Three-Phase Fault13/LConn1 -- Pi Section Line18/LConn1
  DC_14/LConn1 -- DC_12/LConn1 -- DC_1/RConn1
  DC_24/LConn1 -- DC_23/LConn1 -- DC_2/RConn1 -- DC_21/LConn1
  DC_43/LConn1 -- DC_41/LConn1 -- DC_42/LConn1 -- DC_4/LConn1
  Pi Section Line56/RConn1 -- Pi Section Line14/LConn1 -- Three-Phase Fault3/LConn1
  Pi Section Line5/RConn1 -- Three-Phase Fault15/LConn2 -- Pi Section Line57/LConn1
  DC_43/LConn2 -- DC_41/LConn2 -- DC_42/LConn2 -- DC_4/LConn2
  Pi Section Line78/RConn1 -- Three-Phase Fault35/LConn1 -- Pi Section Line76/LConn1
  Pi Section Line72/RConn1 -- Three-Phase Fault33/LConn1 -- Pi Section Line80/LConn1
  Pi Section Line14/RConn1 -- Three-Phase Fault22/LConn1 -- Pi Section Line58/LConn1
  Pi Section Line1/LConn1 -- Pi Section Line27/RConn1 -- Three-Phase Fault1/LConn1
  Pi Section Line44/RConn1 -- Pi Section Line8/LConn1 -- Three-Phase Fault21/LConn1
  DC_3/RConn1 -- DC_34/LConn1 -- DC_32/LConn1
  Pi Section Line19/RConn1 -- Pi Section Line51/LConn1 -- Three-Phase Fault20/LConn2
  Pi Section Line18/RConn1 -- Pi Section Line50/LConn1 -- Three-Phase Fault20/LConn1
  Pi Section Line39/RConn1 -- Pi Section Line29/LConn1
  Pi Section Line35/RConn1 -- Pi Section Line37/LConn1
  Pi Section Line39/LConn1 -- Pi Section Line37/RConn1
  Ideal Switch29/LConn1 -- Pi Section Line31/RConn1
  Pi Section Line31/LConn1 -- Pi Section Line29/RConn1
  Pi Section Line84/RConn1 -- Pi Section Line10/LConn1
  Pi Section Line77/LConn1 -- Pi Section Line79/RConn1
  Ideal Switch11/LConn1 -- DC_43/RConn1
  DC_14/RConn1 -- Ideal Switch20/LConn1
  Pi Section Line83/LConn1 -- Pi Section Line75/RConn1
  Pi Section Line49/LConn1 -- Ideal Switch16/LConn1
  Ideal Switch17/LConn1 -- Pi Section Line48/LConn1
  Ideal Switch33/RConn1 -- Pi Section Line33/LConn1
  Ideal Switch16/RConn1 -- DC_24/RConn2
  Pi Section Line5/LConn1 -- Pi Section Line53/RConn1
  Pi Section Line24/RConn1 -- Pi Section Line26/LConn1
  Ideal Switch17/RConn1 -- DC_24/RConn1
  DC_41/RConn1 -- Ideal Switch4/RConn1
  Pi Section Line20/RConn1 -- Ideal Switch2/LConn1
  Pi Section Line47/LConn1 -- Pi Section Line49/RConn1
  Pi Section Line20/LConn1 -- Pi Section Line10/RConn1
  Pi Section Line78/LConn1 -- Ideal Switch41/LConn1
  DC_14/RConn2 -- Ideal Switch23/LConn1
  Pi Section Line15/LConn1 -- Pi Section Line57/RConn1
  DC_42/RConn2 -- Ideal Switch18/LConn1
  Pi Section Line73/LConn1 -- Three-Phase Fault32/LConn2 -- Pi Section Line77/RConn1
  Pi Section Line53/LConn1 -- Pi Section Line55/RConn1
  DC_32/RConn1 -- Ideal Switch38/RConn1
  Pi Section Line59/LConn1 -- Pi Section Line15/RConn1
  DC_23/RConn1 -- Ideal Switch30/LConn1
  Ideal Switch30/RConn1 -- Pi Section Line32/LConn1
  Pi Section Line58/RConn1 -- Ideal Switch11/RConn1
  Pi Section Line59/RConn1 -- Ideal Switch10/RConn1
  Ideal Switch7/LConn1 -- Pi Section Line55/LConn1
  DC_21/RConn1 -- Ideal Switch41/RConn1
  DC_32/RConn2 -- Ideal Switch29/RConn1
  Pi Section Line45/LConn1 -- Pi Section Line51/RConn1
  Pi Section Line9/RConn1 -- Ideal Switch18/RConn1
  DC_41/RConn2 -- Ideal Switch2/RConn1
  Pi Section Line22/LConn1 -- Ideal Switch23/RConn1
  Ideal Switch7/RConn1 -- DC_34/RConn2
  Pi Section Line8/RConn1 -- Ideal Switch19/RConn1
  Ideal Switch38/LConn1 -- Pi Section Line30/RConn1
  DC_42/RConn1 -- Ideal Switch19/LConn1
  Ideal Switch40/LConn1 -- Pi Section Line79/LConn1
  Pi Section Line11/RConn1 -- Ideal Switch4/LConn1
  DC_23/RConn2 -- Ideal Switch33/LConn1
  Pi Section Line21/LConn1 -- Ideal Switch20/RConn1
  Ideal Switch9/LConn1 -- Pi Section Line54/LConn1
  Pi Section Line9/LConn1 -- Pi Section Line45/RConn1
  Ideal Switch9/RConn1 -- DC_34/RConn1
  Pi Section Line84/LConn1 -- Three-Phase Fault7/LConn2 -- Pi Section Line26/RConn1
  DC_12/RConn1 -- Ideal Switch15/LConn1
  DC_43/RConn2 -- Ideal Switch10/LConn1
  DC_12/RConn2 -- Ideal Switch14/LConn1
  Pi Section Line82/RConn1 -- Ideal Switch15/RConn1
  Pi Section Line75/LConn1 -- Pi Section Line81/RConn1
  Pi Section Line83/RConn1 -- Ideal Switch14/RConn1
  DC_21/RConn2 -- Ideal Switch40/RConn1
  Pi Section Line19/LConn1 -- Pi Section Line47/RConn1

== system clearing_faulted_segment_travelling_Wave/Controlsystem for Inverter ==
  note: Two modes of control:
      | Classical dq0 control
      | Dual sequence dq0 control - allowing negative sequence control
      | such as negative current injection for grid and load support
      | during unbalanced faults.
      |
      | TO CHANGE BETWEEN -> RIGHT CLICK ON THE CONTROL BLOCK OUTSIDE OF THIS SUBSYSTEM
      | -> VARIANT -> OVERRIDE USING
  "I_ph " : Inport
  "V_ph " : Inport  Port=2
  Dq0 Control : Subsystem  VariantControl=Variant1
  Dq0 control with Dual Synchronous Reference Frame (DSRF) : Subsystem  VariantControl=Variant
  " Control Signal1" : Outport

== system clearing_faulted_segment_travelling_Wave/Controlsystem for rectifier ==
  note: Two modes of control:
      | Classical dq0 control
      | Dual sequence dq0 control - allowing negative sequence control
      | such as negative current injection for grid and load support
      | during unbalanced faults.
      |
      | TO CHANGE BETWEEN -> RIGHT CLICK ON THE CONTROL BLOCK OUTSIDE OF THIS SUBSYSTEM
      | -> VARIANT -> OVERRIDE USING
  "I_ph " : Inport
  "V_ph " : Inport  Port=2
  "V_dc " : Inport  Port=3
  Dq0 Control : Subsystem  VariantControl=Variant1
  Dq0 Control with Dual Synchronous Reference Frame (DSRF) : Subsystem  VariantControl=Variant2
  " Control Signal" : Outport
  " wt" : Outport  Port=2

== system clearing_faulted_segment_travelling_Wave/Controlsystem for rectifier1 ==
  note: Two modes of control:
      | Classical dq0 control
      | Dual sequence dq0 control - allowing negative sequence control
      | such as negative current injection for grid and load support
      | during unbalanced faults.
      |
      | TO CHANGE BETWEEN -> RIGHT CLICK ON THE CONTROL BLOCK OUTSIDE OF THIS SUBSYSTEM
      | -> VARIANT -> OVERRIDE USING
  "I_ph " : Inport
  "V_ph " : Inport  Port=2
  "V_dc " : Inport  Port=3
  Dq0 Control : Subsystem  VariantControl=Variant1
  Dq0 Control with Dual Synchronous Reference Frame (DSRF) : Subsystem  VariantControl=Variant2
  " Control Signal" : Outport
  " wt" : Outport  Port=2

== system clearing_faulted_segment_travelling_Wave/Controlsystem for rectifier2 ==
  note: Two modes of control:
      | Classical dq0 control
      | Dual sequence dq0 control - allowing negative sequence control
      | such as negative current injection for grid and load support
      | during unbalanced faults.
      |
      | TO CHANGE BETWEEN -> RIGHT CLICK ON THE CONTROL BLOCK OUTSIDE OF THIS SUBSYSTEM
      | -> VARIANT -> OVERRIDE USING
  "I_ph " : Inport
  "V_ph " : Inport  Port=2
  "V_dc " : Inport  Port=3
  Dq0 Control : Subsystem  VariantControl=Variant1
  Dq0 Control with Dual Synchronous Reference Frame (DSRF) : Subsystem  VariantControl=Variant2
  " Control Signal" : Outport
  " wt" : Outport  Port=2

== system clearing_faulted_segment_travelling_Wave/DC_1 ==
  Current Measurement2 : powerlib/Measurements/Current Measurement  PhasorSimulation=off  OutputType=Complex  PSBequivalent=0
      settings: SourceProductName=Simscape Electrical
  Voltage Measurement1 : powerlib/Measurements/Voltage Measurement  PhasorSimulation=off  OutputType=Complex  PSBequivalent=0
      settings: SourceProductName=Simscape Electrical
  P : PMIOPort  Side=Left
  M : PMIOPort  Port=2  Side=Left
  p : PMIOPort  Port=3  Side=Right
  m : PMIOPort  Port=4  Side=Right
  tag scope: I_dc=global, V_dc=global
  wires:
  Voltage Measurement1/1 -> [V_dc]
  Current Measurement2/1 -> [I_dc]
  connections:
  Current Measurement2/LConn1 -- Voltage Measurement1/LConn1 -- P/RConn1
  Voltage Measurement1/LConn2 -- m/RConn1 -- M/RConn1
  Current Measurement2/RConn1 -- p/RConn1

== system clearing_faulted_segment_travelling_Wave/DC_12 ==
  Current Measurement1 : powerlib/Measurements/Current Measurement  PhasorSimulation=off  OutputType=Complex  PSBequivalent=0
      settings: SourceProductName=Simscape Electrical
  Current Measurement2 : powerlib/Measurements/Current Measurement  PhasorSimulation=off  OutputType=Complex  PSBequivalent=0
      settings: SourceProductName=Simscape Electrical
  Voltage Measurement1 : powerlib/Measurements/Voltage Measurement  PhasorSimulation=off  OutputType=Complex  PSBequivalent=0
      settings: SourceProductName=Simscape Electrical
  P : PMIOPort  Side=Left
  M : PMIOPort  Port=2  Side=Left
  p : PMIOPort  Port=3  Side=Right
  m : PMIOPort  Port=4  Side=Right
  tag scope: I0_dc12=global, I_dc12=global, V_dc12=global
  wires:
  Current Measurement2/1 -> [I_dc12]
  Voltage Measurement1/1 -> [V_dc12]
  Current Measurement1/1 -> [I0_dc12]
  connections:
  Voltage Measurement1/LConn1 -- Current Measurement2/LConn1 -- P/RConn1
  Voltage Measurement1/LConn2 -- M/RConn1 -- Current Measurement1/LConn1
  Current Measurement2/RConn1 -- p/RConn1
  Current Measurement1/RConn1 -- m/RConn1

== system clearing_faulted_segment_travelling_Wave/DC_14 ==
  Current Measurement1 : powerlib/Measurements/Current Measurement  PhasorSimulation=off  OutputType=Complex  PSBequivalent=0
      settings: SourceProductName=Simscape Electrical
  Current Measurement2 : powerlib/Measurements/Current Measurement  PhasorSimulation=off  OutputType=Complex  PSBequivalent=0
      settings: SourceProductName=Simscape Electrical
  Voltage Measurement1 : powerlib/Measurements/Voltage Measurement  PhasorSimulation=off  OutputType=Complex  PSBequivalent=0
      settings: SourceProductName=Simscape Electrical
  P : PMIOPort  Side=Left
  M : PMIOPort  Port=2  Side=Left
  p : PMIOPort  Port=3  Side=Right
  m : PMIOPort  Port=4  Side=Right
  tag scope: I0_dc14=global, I_dc14=global, V_dc14=global
  wires:
  Current Measurement2/1 -> [I_dc14]
  Voltage Measurement1/1 -> [V_dc14]
  Current Measurement1/1 -> [I0_dc14]
  connections:
  Voltage Measurement1/LConn1 -- Current Measurement2/LConn1 -- P/RConn1
  Voltage Measurement1/LConn2 -- Current Measurement1/LConn1 -- M/RConn1
  Current Measurement2/RConn1 -- p/RConn1
  Current Measurement1/RConn1 -- m/RConn1

== system clearing_faulted_segment_travelling_Wave/DC_2 ==
  Current Measurement2 : powerlib/Measurements/Current Measurement  PhasorSimulation=off  OutputType=Complex  PSBequivalent=0
      settings: SourceProductName=Simscape Electrical
  Voltage Measurement1 : powerlib/Measurements/Voltage Measurement  PhasorSimulation=off  OutputType=Complex  PSBequivalent=0
      settings: SourceProductName=Simscape Electrical
  P : PMIOPort  Side=Left
  M : PMIOPort  Port=2  Side=Left
  p : PMIOPort  Port=3  Side=Right
  m : PMIOPort  Port=4  Side=Right
  tag scope: I_dc2=global, V_dc2=global
  wires:
  Voltage Measurement1/1 -> [V_dc2]
  Current Measurement2/1 -> [I_dc2]
  connections:
  Voltage Measurement1/LConn1 -- Current Measurement2/LConn1 -- P/RConn1
  Voltage Measurement1/LConn2 -- M/RConn1 -- m/RConn1
  Current Measurement2/RConn1 -- p/RConn1

== system clearing_faulted_segment_travelling_Wave/DC_21 ==
  Current Measurement1 : powerlib/Measurements/Current Measurement  PhasorSimulation=off  OutputType=Complex  PSBequivalent=0
      settings: SourceProductName=Simscape Electrical
  Current Measurement2 : powerlib/Measurements/Current Measurement  PhasorSimulation=off  OutputType=Complex  PSBequivalent=0
      settings: SourceProductName=Simscape Electrical
  Voltage Measurement1 : powerlib/Measurements/Voltage Measurement  PhasorSimulation=off  OutputType=Complex  PSBequivalent=0
      settings: SourceProductName=Simscape Electrical
  P : PMIOPort  Side=Left
  M : PMIOPort  Port=2  Side=Left
  p : PMIOPort  Port=3  Side=Right
  m : PMIOPort  Port=4  Side=Right
  tag scope: I0_dc21=global, I_dc21=global, V_dc21=global
  wires:
  Current Measurement2/1 -> [I_dc21]
  Voltage Measurement1/1 -> [V_dc21]
  Current Measurement1/1 -> [I0_dc21]
  connections:
  Voltage Measurement1/LConn1 -- Current Measurement2/LConn1 -- P/RConn1
  Voltage Measurement1/LConn2 -- Current Measurement1/LConn1 -- M/RConn1
  Current Measurement2/RConn1 -- p/RConn1
  Current Measurement1/RConn1 -- m/RConn1

== system clearing_faulted_segment_travelling_Wave/DC_23 ==
  Current Measurement1 : powerlib/Measurements/Current Measurement  PhasorSimulation=off  OutputType=Complex  PSBequivalent=0
      settings: SourceProductName=Simscape Electrical
  Current Measurement2 : powerlib/Measurements/Current Measurement  PhasorSimulation=off  OutputType=Complex  PSBequivalent=0
      settings: SourceProductName=Simscape Electrical
  Voltage Measurement1 : powerlib/Measurements/Voltage Measurement  PhasorSimulation=off  OutputType=Complex  PSBequivalent=0
      settings: SourceProductName=Simscape Electrical
  P : PMIOPort  Side=Left
  M : PMIOPort  Port=2  Side=Left
  p : PMIOPort  Port=3  Side=Right
  m : PMIOPort  Port=4  Side=Right
  tag scope: I0_dc23=global, I_dc23=global, V_dc23=global
  wires:
  Current Measurement2/1 -> [I_dc23]
  Voltage Measurement1/1 -> [V_dc23]
  Current Measurement1/1 -> [I0_dc23]
  connections:
  Voltage Measurement1/LConn1 -- Current Measurement2/LConn1 -- P/RConn1
  Current Measurement1/RConn1 -- m/RConn1
  Current Measurement2/RConn1 -- p/RConn1
  Voltage Measurement1/LConn2 -- M/RConn1 -- Current Measurement1/LConn1

== system clearing_faulted_segment_travelling_Wave/DC_24 ==
  Current Measurement1 : powerlib/Measurements/Current Measurement  PhasorSimulation=off  OutputType=Complex  PSBequivalent=0
      settings: SourceProductName=Simscape Electrical
  Current Measurement2 : powerlib/Measurements/Current Measurement  PhasorSimulation=off  OutputType=Complex  PSBequivalent=0
      settings: SourceProductName=Simscape Electrical
  Voltage Measurement1 : powerlib/Measurements/Voltage Measurement  PhasorSimulation=off  OutputType=Complex  PSBequivalent=0
      settings: SourceProductName=Simscape Electrical
  P : PMIOPort  Side=Left
  M : PMIOPort  Port=2  Side=Left
  p : PMIOPort  Port=3  Side=Right
  m : PMIOPort  Port=4  Side=Right
  tag scope: I0_dc24=global, I_dc24=global, V_dc24=global
  wires:
  Current Measurement2/1 -> [I_dc24]
  Voltage Measurement1/1 -> [V_dc24]
  Current Measurement1/1 -> [I0_dc24]
  connections:
  Voltage Measurement1/LConn1 -- Current Measurement2/LConn1 -- P/RConn1
  Voltage Measurement1/LConn2 -- Current Measurement1/LConn1 -- M/RConn1
  Current Measurement2/RConn1 -- p/RConn1
  Current Measurement1/RConn1 -- m/RConn1

== system clearing_faulted_segment_travelling_Wave/DC_3 ==
  Current Measurement2 : powerlib/Measurements/Current Measurement  PhasorSimulation=off  OutputType=Complex  PSBequivalent=0
      settings: SourceProductName=Simscape Electrical
  Voltage Measurement1 : powerlib/Measurements/Voltage Measurement  PhasorSimulation=off  OutputType=Complex  PSBequivalent=0
      settings: SourceProductName=Simscape Electrical
  P : PMIOPort  Side=Left
  M : PMIOPort  Port=2  Side=Left
  p : PMIOPort  Port=3  Side=Right
  m : PMIOPort  Port=4  Side=Right
  tag scope: I_dc3=global, V_dc3=global
  wires:
  Voltage Measurement1/1 -> [V_dc3]
  Current Measurement2/1 -> [I_dc3]
  connections:
  Voltage Measurement1/LConn1 -- Current Measurement2/LConn1 -- P/RConn1
  Voltage Measurement1/LConn2 -- M/RConn1 -- m/RConn1
  Current Measurement2/RConn1 -- p/RConn1

== system clearing_faulted_segment_travelling_Wave/DC_32 ==
  Current Measurement1 : powerlib/Measurements/Current Measurement  PhasorSimulation=off  OutputType=Complex  PSBequivalent=0
      settings: SourceProductName=Simscape Electrical
  Current Measurement2 : powerlib/Measurements/Current Measurement  PhasorSimulation=off  OutputType=Complex  PSBequivalent=0
      settings: SourceProductName=Simscape Electrical
  Voltage Measurement1 : powerlib/Measurements/Voltage Measurement  PhasorSimulation=off  OutputType=Complex  PSBequivalent=0
      settings: SourceProductName=Simscape Electrical
  P : PMIOPort  Side=Left
  M : PMIOPort  Port=2  Side=Left
  p : PMIOPort  Port=3  Side=Right
  m : PMIOPort  Port=4  Side=Right
  tag scope: I0_dc32=global, I_dc32=global, V_dc32=global
  wires:
  Current Measurement2/1 -> [I_dc32]
  Voltage Measurement1/1 -> [V_dc32]
  Current Measurement1/1 -> [I0_dc32]
  connections:
  Voltage Measurement1/LConn1 -- Current Measurement2/LConn1 -- P/RConn1
  Voltage Measurement1/LConn2 -- Current Measurement1/LConn1 -- M/RConn1
  Current Measurement2/RConn1 -- p/RConn1
  Current Measurement1/RConn1 -- m/RConn1

== system clearing_faulted_segment_travelling_Wave/DC_34 ==
  Current Measurement1 : powerlib/Measurements/Current Measurement  PhasorSimulation=off  OutputType=Complex  PSBequivalent=0
      settings: SourceProductName=Simscape Electrical
  Current Measurement2 : powerlib/Measurements/Current Measurement  PhasorSimulation=off  OutputType=Complex  PSBequivalent=0
      settings: SourceProductName=Simscape Electrical
  Voltage Measurement1 : powerlib/Measurements/Voltage Measurement  PhasorSimulation=off  OutputType=Complex  PSBequivalent=0
      settings: SourceProductName=Simscape Electrical
  P : PMIOPort  Side=Left
  M : PMIOPort  Port=2  Side=Left
  p : PMIOPort  Port=3  Side=Right
  m : PMIOPort  Port=4  Side=Right
  tag scope: I0_dc34=global, I_dc34=global, V_dc34=global
  wires:
  Current Measurement2/1 -> [I_dc34]
  Voltage Measurement1/1 -> [V_dc34]
  Current Measurement1/1 -> [I0_dc34]
  connections:
  Voltage Measurement1/LConn1 -- Current Measurement2/LConn1 -- P/RConn1
  Voltage Measurement1/LConn2 -- Current Measurement1/LConn1 -- M/RConn1
  Current Measurement2/RConn1 -- p/RConn1
  Current Measurement1/RConn1 -- m/RConn1

== system clearing_faulted_segment_travelling_Wave/DC_4 ==
  Current Measurement2 : powerlib/Measurements/Current Measurement  PhasorSimulation=off  OutputType=Complex  PSBequivalent=0
      settings: SourceProductName=Simscape Electrical
  Voltage Measurement1 : powerlib/Measurements/Voltage Measurement  PhasorSimulation=off  OutputType=Complex  PSBequivalent=0
      settings: SourceProductName=Simscape Electrical
  P : PMIOPort  Side=Left
  M : PMIOPort  Port=2  Side=Left
  p : PMIOPort  Port=3  Side=Right
  m : PMIOPort  Port=4  Side=Right
  tag scope: I_dc4=global, V_dc4=global
  wires:
  Voltage Measurement1/1 -> [V_dc4]
  Current Measurement2/1 -> [I_dc4]
  connections:
  Voltage Measurement1/LConn1 -- Current Measurement2/LConn1 -- P/RConn1
  Voltage Measurement1/LConn2 -- M/RConn1 -- m/RConn1
  Current Measurement2/RConn1 -- p/RConn1

== system clearing_faulted_segment_travelling_Wave/DC_41 ==
  Current Measurement1 : powerlib/Measurements/Current Measurement  PhasorSimulation=off  OutputType=Complex  PSBequivalent=0
      settings: SourceProductName=Simscape Electrical
  Current Measurement2 : powerlib/Measurements/Current Measurement  PhasorSimulation=off  OutputType=Complex  PSBequivalent=0
      settings: SourceProductName=Simscape Electrical
  Voltage Measurement1 : powerlib/Measurements/Voltage Measurement  PhasorSimulation=off  OutputType=Complex  PSBequivalent=0
      settings: SourceProductName=Simscape Electrical
  P : PMIOPort  Side=Left
  M : PMIOPort  Port=2  Side=Left
  p : PMIOPort  Port=3  Side=Right
  m : PMIOPort  Port=4  Side=Right
  tag scope: I0_dc41=global, I_dc41=global, V_dc41=global
  wires:
  Current Measurement2/1 -> [I_dc41]
  Voltage Measurement1/1 -> [V_dc41]
  Current Measurement1/1 -> [I0_dc41]
  connections:
  Voltage Measurement1/LConn1 -- Current Measurement2/LConn1 -- P/RConn1
  Voltage Measurement1/LConn2 -- Current Measurement1/LConn1 -- M/RConn1
  Current Measurement2/RConn1 -- p/RConn1
  Current Measurement1/RConn1 -- m/RConn1

== system clearing_faulted_segment_travelling_Wave/DC_42 ==
  Current Measurement1 : powerlib/Measurements/Current Measurement  PhasorSimulation=off  OutputType=Complex  PSBequivalent=0
      settings: SourceProductName=Simscape Electrical
  Current Measurement2 : powerlib/Measurements/Current Measurement  PhasorSimulation=off  OutputType=Complex  PSBequivalent=0
      settings: SourceProductName=Simscape Electrical
  Voltage Measurement1 : powerlib/Measurements/Voltage Measurement  PhasorSimulation=off  OutputType=Complex  PSBequivalent=0
      settings: SourceProductName=Simscape Electrical
  P : PMIOPort  Side=Left
  M : PMIOPort  Port=2  Side=Left
  p : PMIOPort  Port=3  Side=Right
  m : PMIOPort  Port=4  Side=Right
  tag scope: I0_dc42=global, I_dc42=global, V_dc42=global
  wires:
  Current Measurement2/1 -> [I_dc42]
  Voltage Measurement1/1 -> [V_dc42]
  Current Measurement1/1 -> [I0_dc42]
  connections:
  Voltage Measurement1/LConn1 -- Current Measurement2/LConn1 -- P/RConn1
  Voltage Measurement1/LConn2 -- Current Measurement1/LConn1 -- M/RConn1
  Current Measurement2/RConn1 -- p/RConn1
  Current Measurement1/RConn1 -- m/RConn1

== system clearing_faulted_segment_travelling_Wave/DC_43 ==
  Current Measurement1 : powerlib/Measurements/Current Measurement  PhasorSimulation=off  OutputType=Complex  PSBequivalent=0
      settings: SourceProductName=Simscape Electrical
  Current Measurement2 : powerlib/Measurements/Current Measurement  PhasorSimulation=off  OutputType=Complex  PSBequivalent=0
      settings: SourceProductName=Simscape Electrical
  Voltage Measurement1 : powerlib/Measurements/Voltage Measurement  PhasorSimulation=off  OutputType=Complex  PSBequivalent=0
      settings: SourceProductName=Simscape Electrical
  P : PMIOPort  Side=Left
  M : PMIOPort  Port=2  Side=Left
  p : PMIOPort  Port=3  Side=Right
  m : PMIOPort  Port=4  Side=Right
  tag scope: I0_dc43=global, I_dc43=global, V_dc43=global
  wires:
  Current Measurement2/1 -> [I_dc43]
  Voltage Measurement1/1 -> [V_dc43]
  Current Measurement1/1 -> [I0_dc43]
  connections:
  Voltage Measurement1/LConn1 -- Current Measurement2/LConn1 -- P/RConn1
  Voltage Measurement1/LConn2 -- Current Measurement1/LConn1 -- M/RConn1
  Current Measurement2/RConn1 -- p/RConn1
  Current Measurement1/RConn1 -- m/RConn1
